simulink model "enabled"  (R2022b)
settings: Solver=ode45  StartTime=0.0  StopTime=10.0  RelTol=1e-3  EnableMultiTasking=on
libraries: simulink x1
settings Model: Creator=nicholas  LastModifiedBy=bensweet
settings SolverCC: AlgebraicLoopSolver=TrustRegion
settings DataIOCC: LimitDataPoints=on  SaveFormat=Array  ReturnWorkspaceOutputs=off  SignalLoggingName=sigsOut
settings OptimizationCC: ExpressionDepthLimit=2147483647  InitFltsAndDblsToZero=on  LifeSpan=inf
settings DebuggingCC: CheckExecutionContextPreStartOutputMsg=on  UnconnectedInputMsg=warning  UnconnectedOutputMsg=warning  UnconnectedLineMsg=warning  PregeneratedLibrarySubsystemCodeDiagnostic=none  SFMachineParentedDataDiag=warning
settings HardwareCC: ProdBitPerPointer=32  ProdBitPerSizeT=32  ProdBitPerPtrDiffT=32  ProdLargestAtomicFloat=None  ProdIntDivRoundTo=Undefined  ProdEndianess=Unspecified  ProdWordSize=32  ProdHWDeviceType=32-bit Generic  TargetUnknown=on
settings ModelReferenceCC: EnableRefExpFcnMdlSchedulingChecks=on  PropagateSignalLabelsOutOfModel=off
settings SFSimCC: SimUseLocalCustomCode=off
settings RTWCC: RTWUseLocalCustomCode=off  DLArmComputeVersion=19.05
settings CodeAppCC: StateflowObjectComments=on
settings GRTTargetCC: TargetFcnLib=ansi_tfl_tmw.mat  TargetLangStandard=C89/C90 (ANSI)  CombineOutputUpdateFcns=off  GRTInterface=on
settings ConfigComp: CovMetricSettings=dw  CovSaveCumulativeToWorkspaceVar=on  CovSaveSingleToWorkspaceVar=on  CovExternalEMLEnable=off  CovSFcnEnable=off

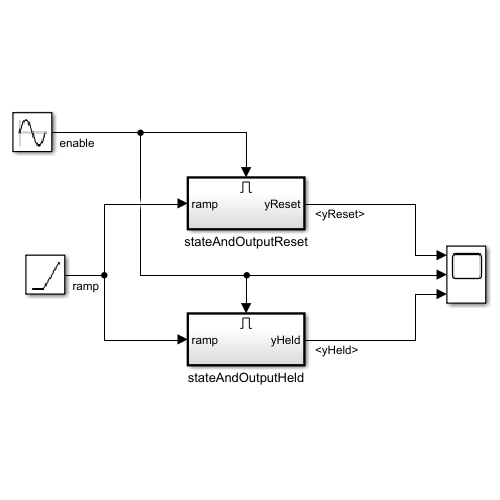
[thumbnail: Simulink's stored preview of the top-level diagram]
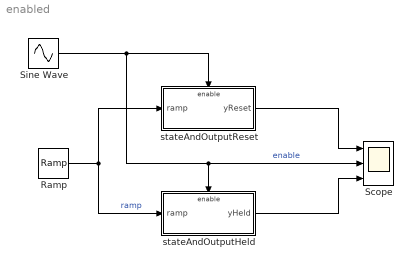
== system enabled ==
  Ramp : simulink/Sources/Ramp  slope=1  start=0  InitialOutput=0
  Scope : Scope  NumInputPorts=3
  Sine Wave : Sin  SampleTime=0
  stateAndOutputHeld : Subsystem  TreatAsAtomicUnit=on
  stateAndOutputReset : Subsystem  TreatAsAtomicUnit=on
  wires:
  Ramp/1 -> stateAndOutputReset/1(ramp), stateAndOutputHeld/1(ramp)  "ramp"
  stateAndOutputHeld/1(yHeld) -> Scope/3
  stateAndOutputReset/1(yReset) -> Scope/1
  Sine Wave/1 -> stateAndOutputHeld/Enable, Scope/2, stateAndOutputReset/Enable  "enable"

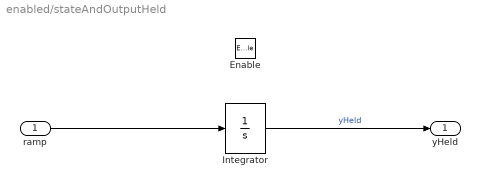
== system enabled/stateAndOutputHeld ==
  ramp : Inport
  Enable : EnablePort
      settings: AttributesFormatString=States when enabling: %<StatesWhenEnabling>
  Integrator : Integrator
  yHeld : Outport  InitialOutput=0  VectorParamsAs1DForOutWhenUnconnected=off
      settings: AttributesFormatString="Output when\\ndisabled:  %<OutputWhenDisabled>"
  wires:
  ramp/1 -> Integrator/1
  Integrator/1 -> yHeld/1  "yHeld"

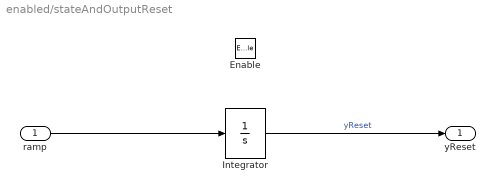
== system enabled/stateAndOutputReset ==
  ramp : Inport
  Enable : EnablePort  StatesWhenEnabling=reset
      settings: AttributesFormatString=States when enabling: %<StatesWhenEnabling>
  Integrator : Integrator
  yReset : Outport  OutputWhenDisabled=reset  InitialOutput=0  VectorParamsAs1DForOutWhenUnconnected=off
      settings: AttributesFormatString="Output when\\ndisabled:  %<OutputWhenDisabled>"
  wires:
  Integrator/1 -> yReset/1  "yReset"
  ramp/1 -> Integrator/1
